simulink model "sampleModel1398"  (R2023a)
settings: Solver=VariableStepAuto  StartTime=0.0  StopTime=10.0  RelTol=1e-3
libraries: hdlsllib x6
settings Model: Creator=user1  LastModifiedBy=user1

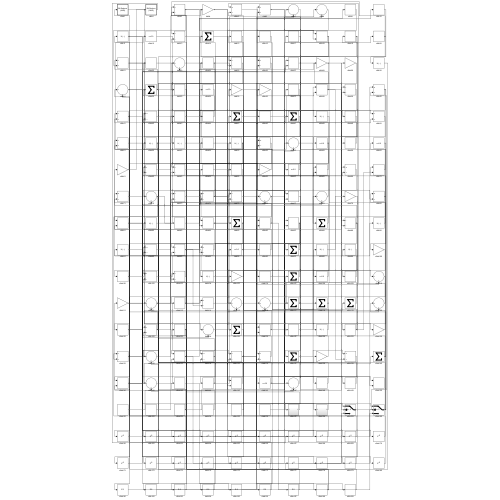
[thumbnail: Simulink's stored preview of the top-level diagram]
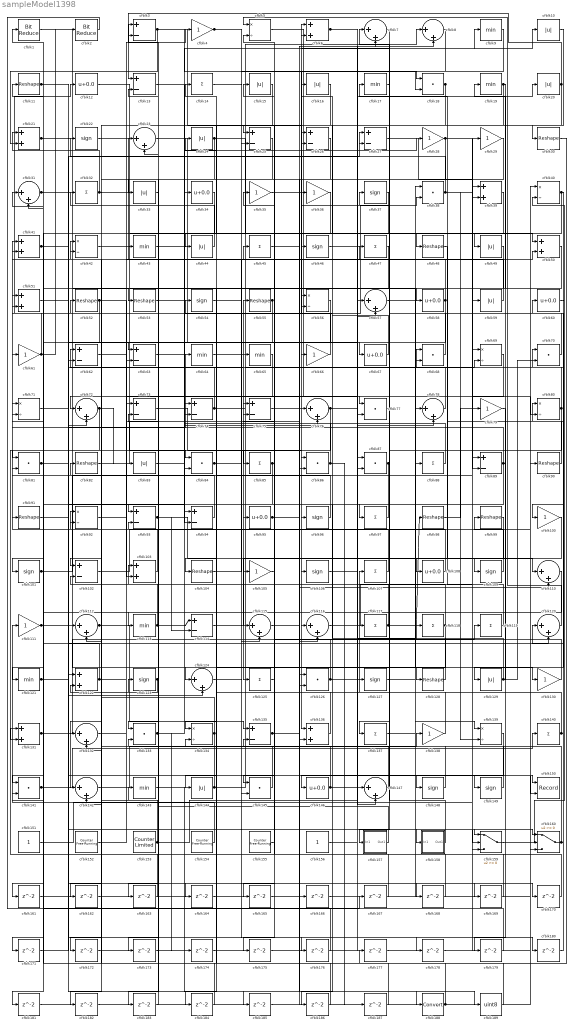
== system sampleModel1398 ==
  cfblk1 : hdlsllib/Logic and Bit Operations/Bit Reduce  mode=AND
  cfblk{10,15..16,20,24,33,44,49,59,83,129,144} (12 alike) : Abs  SaturateOnIntegerOverflow=off
  cfblk{4,28..29,35..36,61,66,79,100,105,111,130,138} (13 alike) : Gain
  cfblk{22,37,46,54,96,101,106,109,123,127,148..149} (12 alike) : Signum
  cfblk{3,13,25..27,62..63,73..75,89,93..94,102,114,135} (16 alike) : Sum  Inputs=+-
  cfblk{6,21,39,41,50..51,103,122,131,136} (10 alike) : Sum
  cfblk{11,30,48,52..53,55,82,90..91,98..99,104,128} (13 alike) : Reshape
  cfblk{14,32,45,47,85,88,97,107,117..119,125,137,140} (14 alike) : Sum  Inputs=+
  cfblk{12,34,58,60,67,95,108,146} (8 alike) : Bias  Bias=0.0  SaturateOnIntegerOverflow=off
  cfblk{7..8,23,31,57,72,76,78,110,112,115..116,120,124,132,142,147} (17 alike) : Sum  Inputs=|++
  cfblk{9,17,19,43,64..65,113,121,143} (9 alike) : MinMax
  cfblk{18,38,68,70,77,81,84,86..87,126,133,141,145} (13 alike) : DotProduct  OutDataTypeStr=Inherit: Inherit via internal rule
  cfblk{5,40,42,56,69,71,80,92,134,139} (10 alike) : Product  Inputs=*/  RndMeth=Zero  SaturateOnIntegerOverflow=on
  cfblk150 : Record  FileSettingsInternal="{\"entries\":[{\"content\":{\"excelSettings\":{\"content\":{},\"type\":\"Streamout.ExcelSettings\"}},\"type\":\"Streamout.FileSettingStorage\",\"uuid\":\"\"}],\"packageUris\":[\"http:\\/\\/schema.mathworks.com\\/mf0\\/streamout_blocks\\/R2020a\"],\"version\":\"1.0\"}"  Layout=[1 1]  SignalsInternal="{\"entries\":[{\"content\":{\"signals\":[{\"content\":{\"blockPath\":[],\"dimensions\":[1],\"domain\":\"\",\"lineColor\":\"#a2142f\",\"plots\":[1],\"port\":1,\"signalID\":88,\"signalName\":\"XY Graph:1\"},\"type\":\"RecordBlkView.Signal\",\"uuid\":\"\"},{\"content\":{\"blockPath\":[],\"dimensions\":[1],\"domain\":\"\",\"lineColor\":\"#139fff\",\"plots\":[1],\"port\":2,\"signalID\":91,\"signalName\":\"XY Graph:2\"},\"type\":\"RecordBlkView.Signal\",\"uuid\":\"\"}]},\"type\":\"RecordBlkView.InputSignals\",\"uuid\":\"\"}],\"packageUris\":[\"http:\\/\\/schema.mathworks.com\\/mf0\\/streamout_blocks\\/R2020a\"],\"version\":\"1.0\"}"  VisualizationBindings="{\"xyplotplugin\":{\"info\":[{\"series\":[{\"bindingParametersList\":[{\"parameter\":\"X-Axis\",\"signalID\":88,\"signalName\":\"XY Graph:1\"},{\"parameter\":\"Y-Axis\",\"signalID\":91,\"signalName\":\"XY Graph:2\"}],\"seriesID\":42092}],\"subplotID\":1}]}}"  CompatibilityTag=XY  st=-1
  cfblk151 : Constant  SampleTime=-1
  cfblk152 : hdlsllib/Sources/Counter Free-Running  NumBits=16  tsamp=-1
  cfblk153 : hdlsllib/Sources/Counter Limited  uplimit=7  tsamp=-1
  cfblk154 : hdlsllib/Sources/Counter Free-Running  NumBits=16  tsamp=-1
  cfblk155 : hdlsllib/Sources/Counter Free-Running  NumBits=16  tsamp=-1
  cfblk156 : Constant  SampleTime=-1
  cfblk157 : Subsystem
      settings: LibrarySourceBlock=|
      | hdlsllib/Ports &
      | Subsystems/Subsystem
  cfblk158 : Subsystem
      settings: LibrarySourceBlock=|
      | hdlsllib/Ports &
      | Subsystems/Subsystem
  cfblk159 : Switch  SaturateOnIntegerOverflow=off  InputSameDT=off
  cfblk160 : Switch  SaturateOnIntegerOverflow=off  InputSameDT=off
  cfblk{161..187} (27 alike) : Delay  SampleTime=1
  cfblk188 : DataTypeConversion  SaturateOnIntegerOverflow=off  RndMeth=Floor
  cfblk189 : DataTypeConversion  OutDataTypeStr=uint8  SaturateOnIntegerOverflow=off  RndMeth=Floor
  cfblk2 : hdlsllib/Logic and Bit Operations/Bit Reduce  mode=AND
  wires:
  cfblk39/1 -> cfblk136/1
  cfblk98/1 -> cfblk79/1
  cfblk19/1 -> cfblk58/1, cfblk67/1
  cfblk42/1 -> cfblk84/1
  cfblk140/1 -> cfblk107/1, cfblk70/1
  cfblk141/1 -> cfblk140/1, cfblk27/2, cfblk72/2
  cfblk1/1 -> cfblk124/1
  cfblk144/1 -> cfblk8/1, cfblk13/2
  cfblk31/1 -> cfblk128/1, cfblk94/2
  cfblk86/1 -> cfblk64/1, cfblk187/1
  cfblk154/1 -> cfblk111/1
  cfblk23/1 -> cfblk116/1
  cfblk65/1 -> cfblk84/2
  cfblk120/1 -> cfblk5/1
  cfblk81/1 -> cfblk74/2, cfblk168/1
  cfblk97/1 -> cfblk93/1
  cfblk22/1 -> cfblk50/1
  cfblk106/1 -> cfblk150/1
  cfblk108/1 -> cfblk7/1
  cfblk56/1 -> cfblk63/1
  cfblk114/1 -> cfblk55/1
  cfblk93/1 -> cfblk106/1, cfblk9/1, cfblk114/2
  cfblk17/1 -> cfblk157/1(In1)
  cfblk117/1 -> cfblk98/1, cfblk75/2
  cfblk61/1 -> cfblk12/1, cfblk2/1
  cfblk116/1 -> cfblk29/1
  cfblk64/1 -> cfblk38/2
  cfblk8/1 -> cfblk96/1
  cfblk12/1 -> cfblk117/1
  cfblk28/1 -> cfblk133/1, cfblk80/2
  cfblk105/1 -> cfblk5/2
  cfblk158/1(Out1) -> cfblk74/1
  cfblk107/1 -> cfblk41/1
  cfblk99/1 -> cfblk125/1
  cfblk145/1 -> cfblk24/1
  cfblk134/1 -> cfblk142/1, cfblk92/2
  cfblk66/1 -> cfblk6/1
  cfblk20/1 -> cfblk13/1, cfblk85/1
  cfblk3/1 -> cfblk115/1, cfblk18/2, cfblk21/2
  cfblk96/1 -> cfblk54/1
  cfblk77/1 -> cfblk97/1
  cfblk72/1 -> cfblk121/1, cfblk83/1
  cfblk24/1 -> cfblk48/1, cfblk72/1
  cfblk58/1 -> cfblk23/1, cfblk62/2, cfblk103/2
  cfblk60/1 -> cfblk129/1
  cfblk43/1 -> cfblk147/1
  cfblk57/1 -> cfblk130/1
  cfblk148/1 -> cfblk82/1
  cfblk101/1 -> cfblk39/1, cfblk71/1
  cfblk155/1 -> cfblk105/1
  cfblk135/1 -> cfblk8/2, cfblk159/1
  cfblk131/1 -> cfblk119/1, cfblk120/2
  cfblk21/1 -> cfblk53/1, cfblk178/1
  cfblk100/1 -> cfblk145/1
  cfblk53/1 -> cfblk10/1
  cfblk159/1 -> cfblk40/2
  cfblk27/1 -> cfblk89/1
  cfblk115/1 -> cfblk149/1
  cfblk54/1 -> cfblk150/2
  cfblk112/1 -> cfblk135/1, cfblk75/1
  cfblk136/1 -> cfblk35/1
  cfblk44/1 -> cfblk32/1
  cfblk138/1 -> cfblk91/1
  cfblk151/1 -> cfblk39/2
  cfblk16/1 -> cfblk102/1
  cfblk146/1 -> cfblk20/1, cfblk78/2, cfblk92/1
  cfblk40/1 -> cfblk100/1, cfblk81/1
  cfblk76/1 -> cfblk127/1, cfblk131/2
  cfblk103/1 -> cfblk11/1
  cfblk88/1 -> cfblk14/1
  cfblk55/1 -> cfblk51/2, cfblk163/1
  cfblk118/1 -> cfblk134/1, cfblk42/2
  cfblk15/1 -> cfblk25/1
  cfblk149/1 -> cfblk37/1
  cfblk128/1 -> cfblk52/1
  cfblk133/1 -> cfblk34/1, cfblk174/1
  cfblk46/1 -> cfblk49/1
  cfblk35/1 -> cfblk87/2
  cfblk113/1 -> cfblk114/1, cfblk102/2, cfblk56/1
  cfblk29/1 -> cfblk126/2
  cfblk84/1 -> cfblk115/2, cfblk158/1(In1)
  cfblk13/1 -> cfblk76/2
  cfblk69/1 -> cfblk132/1
  cfblk142/1 -> cfblk138/1
  cfblk32/1 -> cfblk88/1, cfblk21/1, cfblk142/2
  cfblk85/1 -> cfblk15/1, cfblk104/1
  cfblk156/1 -> cfblk118/1
  cfblk33/1 -> cfblk113/1
  cfblk25/1 -> cfblk33/1
  cfblk49/1 -> cfblk89/2
  cfblk160/1 -> cfblk60/1, cfblk42/1, cfblk80/1
  cfblk79/1 -> cfblk109/1
  cfblk5/1 -> cfblk147/2
  cfblk123/1 -> cfblk122/2, cfblk183/1
  cfblk6/1 -> cfblk18/1, cfblk148/1
  cfblk87/1 -> cfblk146/1, cfblk184/1
  cfblk157/1(Out1) -> cfblk123/1
  cfblk147/1 -> cfblk112/2
  cfblk132/1 -> cfblk73/1
  cfblk73/1 -> cfblk86/1
  cfblk152/1 -> cfblk43/1
  cfblk80/1 -> cfblk137/1, cfblk3/1
  cfblk94/1 -> cfblk61/1
  cfblk143/1 -> cfblk188/1
  cfblk153/1 -> cfblk28/1, cfblk51/1
  cfblk38/1 -> cfblk59/1, cfblk22/1, cfblk139/2
  cfblk92/1 -> cfblk4/1
  cfblk68/1 -> cfblk36/1
  cfblk9/1 -> cfblk25/2
  cfblk18/1 -> cfblk44/1, cfblk46/1
  cfblk90/1 -> cfblk17/1
  cfblk122/1 -> cfblk63/2, cfblk81/2, cfblk182/1
  cfblk48/1 -> cfblk108/1
  cfblk11/1 -> cfblk145/2, cfblk66/1
  cfblk121/1 -> cfblk65/1, cfblk26/2
  cfblk126/1 -> cfblk69/2, cfblk103/1
  cfblk102/1 -> cfblk90/1
  cfblk129/1 -> cfblk19/1, cfblk70/2, cfblk56/2
  cfblk4/1 -> cfblk110/1, cfblk26/1
  cfblk47/1 -> cfblk144/1
  cfblk124/1 -> cfblk160/1
  cfblk70/1 -> cfblk6/2
  cfblk74/1 -> cfblk57/1, cfblk3/2, cfblk169/1
  cfblk10/1 -> cfblk30/1
  cfblk127/1 -> cfblk78/1
  cfblk7/1 -> cfblk77/1
  cfblk41/1 -> cfblk101/1, cfblk185/1
  cfblk82/1 -> cfblk68/1
  cfblk119/1 -> cfblk68/2
  cfblk95/1 -> cfblk45/1, cfblk110/2
  cfblk111/1 -> cfblk124/2, cfblk159/2
  cfblk63/1 -> cfblk94/1
  cfblk62/1 -> cfblk50/2
  cfblk67/1 -> cfblk16/1
  cfblk52/1 -> cfblk141/1, cfblk77/2
  cfblk59/1 -> cfblk31/1
  cfblk83/1 -> cfblk27/1
  cfblk109/1 -> cfblk99/1
  cfblk104/1 -> cfblk47/1
  cfblk130/1 -> cfblk95/1
  cfblk137/1 -> cfblk139/1
  cfblk89/1 -> cfblk71/2, cfblk179/1, cfblk181/1
  cfblk78/1 -> cfblk62/1
  cfblk50/1 -> cfblk161/1
  cfblk161/1 -> cfblk76/1
  cfblk36/1 -> cfblk162/1
  cfblk162/1 -> cfblk160/2
  cfblk163/1 -> cfblk41/2
  cfblk51/1 -> cfblk164/1
  cfblk164/1 -> cfblk38/1
  cfblk125/1 -> cfblk165/1
  cfblk165/1 -> cfblk126/1
  cfblk75/1 -> cfblk166/1
  cfblk166/1 -> cfblk7/2
  cfblk2/1 -> cfblk167/1
  cfblk167/1 -> cfblk135/2
  cfblk168/1 -> cfblk87/1
  cfblk169/1 -> cfblk131/1
  cfblk91/1 -> cfblk170/1
  cfblk170/1 -> cfblk1/1
  cfblk110/1 -> cfblk171/1
  cfblk171/1 -> cfblk112/1
  cfblk26/1 -> cfblk172/1
  cfblk172/1 -> cfblk136/2
  cfblk34/1 -> cfblk173/1
  cfblk173/1 -> cfblk23/2
  cfblk174/1 -> cfblk57/2
  cfblk37/1 -> cfblk175/1
  cfblk175/1 -> cfblk40/1
  cfblk14/1 -> cfblk176/1
  cfblk176/1 -> cfblk122/1
  cfblk30/1 -> cfblk177/1
  cfblk177/1 -> cfblk69/1
  cfblk178/1 -> cfblk159/3
  cfblk179/1 -> cfblk31/2
  cfblk71/1 -> cfblk180/1
  cfblk180/1 -> cfblk120/1
  cfblk181/1 -> cfblk86/2
  cfblk182/1 -> cfblk116/2
  cfblk183/1 -> cfblk93/2
  cfblk184/1 -> cfblk141/2
  cfblk185/1 -> cfblk160/3
  cfblk139/1 -> cfblk186/1
  cfblk186/1 -> cfblk73/2
  cfblk187/1 -> cfblk132/2
  cfblk188/1 -> cfblk133/2, cfblk134/2
  cfblk45/1 -> cfblk189/1
  cfblk189/1 -> cfblk143/1

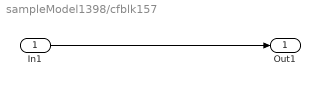
== system sampleModel1398/cfblk157 ==
  In1 : Inport
  Out1 : Outport
  wires:
  In1/1 -> Out1/1

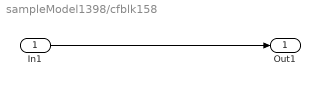
== system sampleModel1398/cfblk158 ==
  In1 : Inport
  Out1 : Outport
  wires:
  In1/1 -> Out1/1
